simulink model "IHC_NL_Logarithmic_Function"  (R2019b)
settings: Solver=VariableStepAuto  StartTime=0.0  StopTime=testtime  RelTol=1e-3
InitFcn:
  | IHC_NL_Logarithmic_Test_Parameters
StopFcn:
  | Verify_IHC_NL_Logarithmic_Function
values from neighbouring files (symbols this model uses):
  Fs = 48e3    (= 48000)    [IHC_NL_Logarithmic_Test_Parameters.m]
  ihcasym = 3.0    (= 3)    [IHC_NL_Logarithmic_Test_Parameters.m]
  slope = 0.1    [IHC_NL_Logarithmic_Test_Parameters.m]
  strength = (20.0e6)/(10^(corner/20))    (= 2000)    [IHC_NL_Logarithmic_Test_Parameters.m]
libraries: dspsrcs4 x2, simulink x1
settings Model: Creator=mblun  LastModifiedBy=t96f346
settings OptimizationCC: BlockReduction=off  ConditionallyExecuteInputs=off  DefaultParameterBehavior=Inlined
settings DebuggingCC: AlgebraicLoopMsg=error
settings HardwareCC: ProdBitPerPointer=32  ProdBitPerSizeT=32  ProdBitPerPtrDiffT=32  ProdLargestAtomicFloat=None  ProdIntDivRoundTo=Undefined  ProdEndianess=Unspecified  ProdWordSize=32  ProdHWDeviceType=ASIC/FPGA->ASIC/FPGA  TargetBitPerPointer=64  TargetBitPerSizeT=64  TargetBitPerPtrDiffT=64  TargetLongLongMode=on  TargetIntDivRoundTo=Zero  TargetEndianess=LittleEndian  TargetWordSize=64  TargetHWDeviceType=Custom Processor->MATLAB Host Computer  ProdEqTarget=off
settings SFSimCC: CustomCodeUndefinedFunction=UseInterfaceOnly

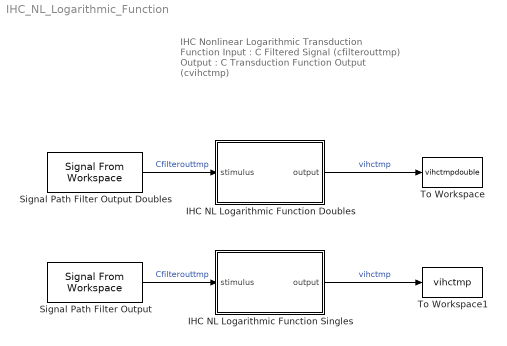
== system IHC_NL_Logarithmic_Function ==
  note: IHC Nonlinear Logarithmic Transduction Function
      |
      | Input : C Filtered Signal (cfilterouttmp)
      |
      | Output : C Transduction Function Output (cvihctmp)
  IHC NL Logarithmic Function Doubles : Subsystem
  IHC NL Logarithmic Function Singles : Subsystem
  Signal Path Filter Output : dspsrcs4/Signal From Workspace  X=RxSignal  Ts=1/Fs  nsamps=1  OutputAfterFinalValue=Setting to zero  ignoreOrWarnInputAndFrameLengths=off  OutputFrames=off
  Signal Path Filter Output Doubles : dspsrcs4/Signal From Workspace  X=RxSignalDouble  Ts=1/Fs  nsamps=1  OutputAfterFinalValue=Setting to zero  ignoreOrWarnInputAndFrameLengths=off  OutputFrames=off
  To Workspace : ToWorkspace  VariableName=vihctmpdouble  SampleTime=-1
      settings: Save2DSignal=2-D array (concatenate along first dimension)
  To Workspace1 : ToWorkspace  VariableName=vihctmp  SampleTime=-1
      settings: Save2DSignal=2-D array (concatenate along first dimension)
  wires:
  Signal Path Filter Output Doubles/1 -> IHC NL Logarithmic Function Doubles/1(stimulus)  "Cfilterouttmp"
  IHC NL Logarithmic Function Doubles/1(output) -> To Workspace/1  "vihctmp"
  Signal Path Filter Output/1 -> IHC NL Logarithmic Function Singles/1(stimulus)  "Cfilterouttmp"
  IHC NL Logarithmic Function Singles/1(output) -> To Workspace1/1  "vihctmp"

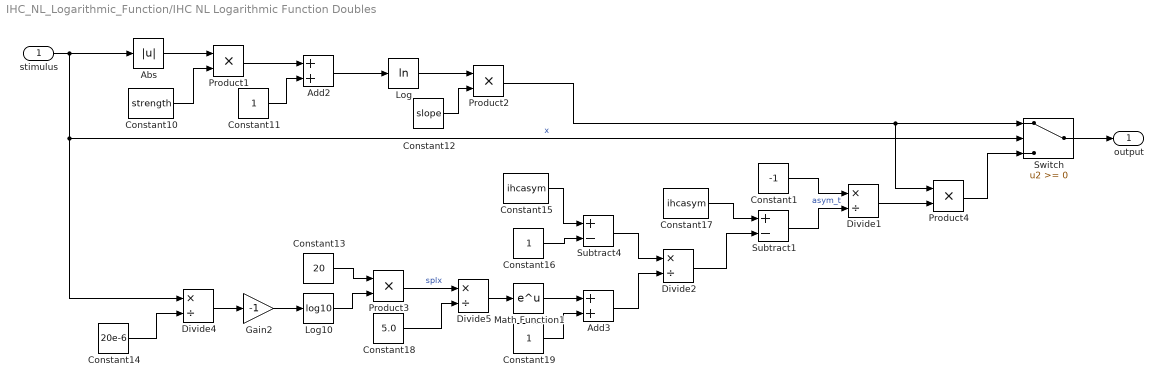
== system IHC_NL_Logarithmic_Function/IHC NL Logarithmic Function Doubles ==
  stimulus : Inport
  Abs : Abs
  Add2 : Sum
  Add3 : Sum
  Constant1 : Constant  Value=-1  SampleTime=-1
  Constant10 : Constant  Value=strength  SampleTime=-1
  Constant11 : Constant  SampleTime=-1
  Constant12 : Constant  Value=slope  SampleTime=-1
  Constant13 : Constant  Value=20  SampleTime=-1
  Constant14 : Constant  Value=20e-6  SampleTime=-1
  Constant15 : Constant  Value=ihcasym  SampleTime=-1
  Constant16 : Constant  SampleTime=-1
  Constant17 : Constant  Value=ihcasym  SampleTime=-1
  Constant18 : Constant  Value=5.0  SampleTime=-1
  Constant19 : Constant  SampleTime=-1
  Divide{1..2,4..5} (4 alike) : Product  Inputs=*/  SaturateOnIntegerOverflow=on  RndMeth=Zero
  Gain2 : Gain  Gain=-1
  Log : Math  Operator=log  SaturateOnIntegerOverflow=on
  Log10 : Math  Operator=log10  SaturateOnIntegerOverflow=on
  Math Function1 : Math  SaturateOnIntegerOverflow=on
  Product{1..4} (4 alike) : Product
  Subtract1 : Sum  Inputs=+-
  Subtract4 : Sum  Inputs=+-
  Switch : Switch
  output : Outport  VectorParamsAs1DForOutWhenUnconnected=off
  wires:
  stimulus/1 -> Divide4/1, Switch/2, Abs/1  "x"
  Abs/1 -> Product1/1
  Constant10/1 -> Product1/2
  Constant11/1 -> Add2/2
  Product1/1 -> Add2/1
  Add2/1 -> Log/1
  Log/1 -> Product2/1
  Constant12/1 -> Product2/2
  Product2/1 -> Product4/1, Switch/1
  Constant14/1 -> Divide4/2
  Divide4/1 -> Gain2/1
  Gain2/1 -> Log10/1
  Log10/1 -> Product3/2
  Constant13/1 -> Product3/1
  Product3/1 -> Divide5/1  "splx"
  Constant15/1 -> Subtract4/1
  Constant16/1 -> Subtract4/2
  Constant18/1 -> Divide5/2
  Divide5/1 -> Math Function1/1
  Math Function1/1 -> Add3/1
  Constant19/1 -> Add3/2
  Subtract4/1 -> Divide2/1
  Add3/1 -> Divide2/2
  Constant17/1 -> Subtract1/1
  Divide2/1 -> Subtract1/2
  Subtract1/1 -> Divide1/2  "asym_t"
  Constant1/1 -> Divide1/1
  Divide1/1 -> Product4/2
  Product4/1 -> Switch/3
  Switch/1 -> output/1

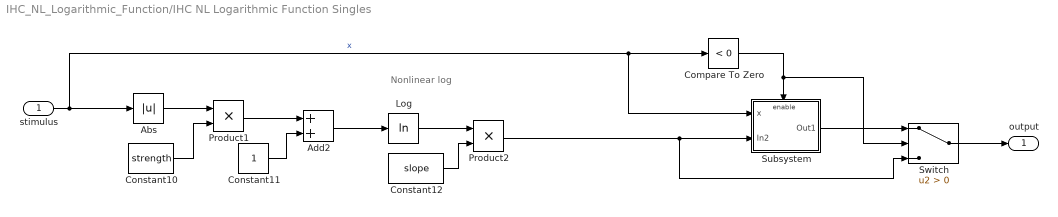
== system IHC_NL_Logarithmic_Function/IHC NL Logarithmic Function Singles ==
  note: Nonlinear log
  stimulus : Inport
  Abs : Abs
  Add2 : Sum
  Compare To Zero : simulink/Logic and Bit Operations/Compare To Zero  relop=<  OutDataTypeStr=boolean
  Constant10 : Constant  Value=strength  OutDataTypeStr=single  SampleTime=-1
  Constant11 : Constant  OutDataTypeStr=single  SampleTime=-1
  Constant12 : Constant  Value=slope  OutDataTypeStr=single  SampleTime=-1
  Log : Math  Operator=log  SaturateOnIntegerOverflow=on
  Product1 : Product
  Product2 : Product
  Subsystem : Subsystem
  Switch : Switch  Criteria=u2 > Threshold
  output : Outport  VectorParamsAs1DForOutWhenUnconnected=off
  wires:
  stimulus/1 -> Subsystem/1(x), Compare To Zero/1, Abs/1  "x"
  Abs/1 -> Product1/1
  Constant10/1 -> Product1/2
  Constant11/1 -> Add2/2
  Product1/1 -> Add2/1
  Add2/1 -> Log/1
  Log/1 -> Product2/1
  Constant12/1 -> Product2/2
  Product2/1 -> Switch/3, Subsystem/2(In2)
  Compare To Zero/1 -> Subsystem/Enable, Switch/2
  Subsystem/1(Out1) -> Switch/1
  Switch/1 -> output/1

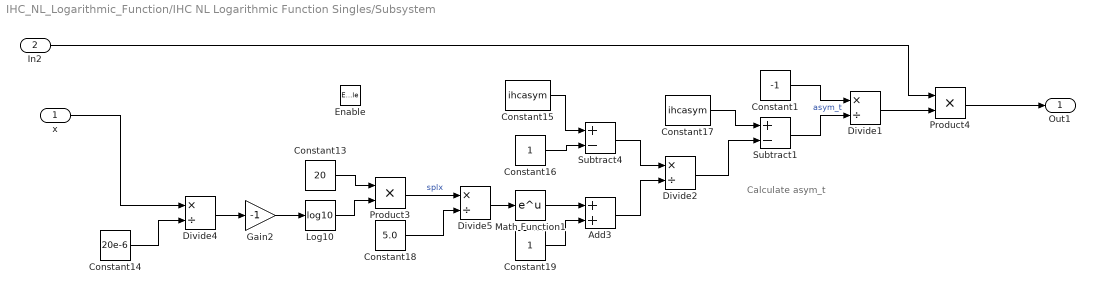
== system IHC_NL_Logarithmic_Function/IHC NL Logarithmic Function Singles/Subsystem ==
  note: Calculate asym_t
  x : Inport
  In2 : Inport  Port=2
  Enable : EnablePort
  Add3 : Sum
  Constant1 : Constant  Value=-1  OutDataTypeStr=single  SampleTime=-1
  Constant13 : Constant  Value=20  OutDataTypeStr=single  SampleTime=-1
  Constant14 : Constant  Value=20e-6  OutDataTypeStr=single  SampleTime=-1
  Constant15 : Constant  Value=ihcasym  OutDataTypeStr=single  SampleTime=-1
  Constant16 : Constant  OutDataTypeStr=single  SampleTime=-1
  Constant17 : Constant  Value=ihcasym  OutDataTypeStr=single  SampleTime=-1
  Constant18 : Constant  Value=5.0  OutDataTypeStr=single  SampleTime=-1
  Constant19 : Constant  OutDataTypeStr=single  SampleTime=-1
  Divide{1..2,4..5} (4 alike) : Product  Inputs=*/  SaturateOnIntegerOverflow=on  RndMeth=Zero
  Gain2 : Gain  Gain=-1
  Log10 : Math  Operator=log10  SaturateOnIntegerOverflow=on
  Math Function1 : Math  SaturateOnIntegerOverflow=on
  Product3 : Product
  Product4 : Product
  Subtract1 : Sum  Inputs=+-
  Subtract4 : Sum  Inputs=+-
  Out1 : Outport  OutDataTypeStr=single  InitialOutput=[0]
  wires:
  Gain2/1 -> Log10/1
  Constant13/1 -> Product3/1
  Divide5/1 -> Math Function1/1
  Math Function1/1 -> Add3/1
  Product3/1 -> Divide5/1  "splx"
  Constant15/1 -> Subtract4/1
  Log10/1 -> Product3/2
  Constant14/1 -> Divide4/2
  Constant19/1 -> Add3/2
  Divide4/1 -> Gain2/1
  Constant18/1 -> Divide5/2
  Subtract4/1 -> Divide2/1
  Constant17/1 -> Subtract1/1
  Add3/1 -> Divide2/2
  Divide2/1 -> Subtract1/2
  Subtract1/1 -> Divide1/2  "asym_t"
  Constant1/1 -> Divide1/1
  Constant16/1 -> Subtract4/2
  Divide1/1 -> Product4/2
  In2/1 -> Product4/1
  x/1 -> Divide4/1
  Product4/1 -> Out1/1
